simulink model "dsogi_pll_arch"  (R2023a)
settings: Solver=VariableStepAuto  StartTime=0.0  StopTime=10.0  RelTol=1e-3
settings Model: DataDictionary=dictionary.sldd  Creator=ASUSTUF  LastModifiedBy=ASUSTUF

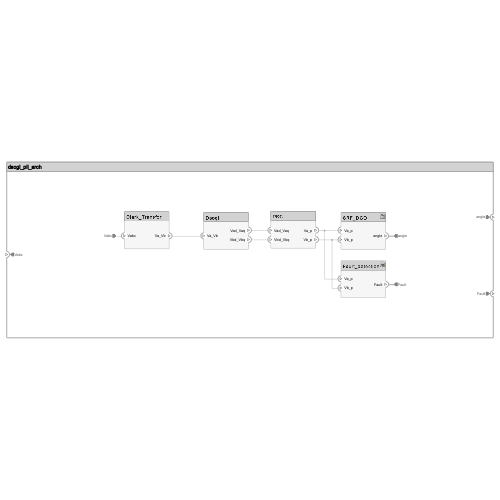
[thumbnail: Simulink's stored preview of the top-level diagram]
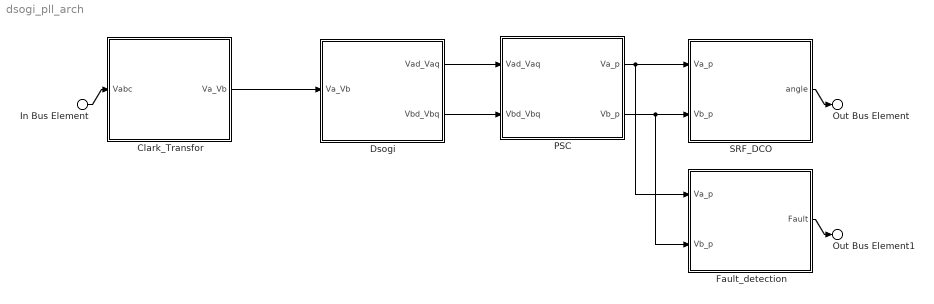
== system dsogi_pll_arch ==
  In Bus Element : Inport  PortName=Vabc
  Clark_Transfor : Subsystem
      settings: PortSchema="{\"entries\":[{\"content\":{\"headerSize\":26,\"margin\":15,\"minimumSpacing\":25,\"sides\":[{\"content\":{\"connectorIds\":[\"In1\"]},\"type\":\"ConnectorPlacement.EquallySpacedRectSide\",\"uuid\":\"d98255bb-0e2e-436f-ac53-b41bd6cffae4\"},{\"content\":{\"connectorIds\":[\"Out1\"],\"side\":\"RIGHT\"},\"type\":\"ConnectorPlacement.EquallySpacedRectSide\",\"uuid\":\"38fda810-9180-46c2-b72f-a00921e55bae\"},{\"content\":{\"side\":\"TOP\"},\"type\":\"ConnectorPlacement.EquallySpacedRectSide\",\"uuid\":\"74ae08d3-cfde-4772-a14d-4780a47b2df7\"}]},\"type\":\"ConnectorPlacement.EquallySpacedConnector\",\"uuid\":\"be157ddc-8a55-4c3c-90ba-55b865cce77e\"}],\"packageUris\":[\"http://schema.mathworks.com/mf0/Connector/R2020b\"],\"version\":\"1.0\"}"
  Dsogi : Subsystem
      settings: PortSchema="{\"entries\":[{\"content\":{\"headerSize\":26,\"margin\":15,\"minimumSpacing\":25,\"sides\":[{\"content\":{\"connectorIds\":[\"In1\"]},\"type\":\"ConnectorPlacement.EquallySpacedRectSide\",\"uuid\":\"d98255bb-0e2e-436f-ac53-b41bd6cffae4\"},{\"content\":{\"connectorIds\":[\"Out1\",\"Out2\"],\"side\":\"RIGHT\"},\"type\":\"ConnectorPlacement.EquallySpacedRectSide\",\"uuid\":\"38fda810-9180-46c2-b72f-a00921e55bae\"},{\"content\":{\"side\":\"TOP\"},\"type\":\"ConnectorPlacement.EquallySpacedRectSide\",\"uuid\":\"74ae08d3-cfde-4772-a14d-4780a47b2df7\"}]},\"type\":\"ConnectorPlacement.EquallySpacedConnector\",\"uuid\":\"be157ddc-8a55-4c3c-90ba-55b865cce77e\"}],\"packageUris\":[\"http://schema.mathworks.com/mf0/Connector/R2020b\"],\"version\":\"1.0\"}"
  Fault_detection : Subsystem
      settings: PortSchema="{\"entries\":[{\"content\":{\"headerSize\":26,\"margin\":15,\"minimumSpacing\":25,\"sides\":[{\"content\":{\"connectorIds\":[\"In1\",\"In2\"]},\"type\":\"ConnectorPlacement.EquallySpacedRectSide\",\"uuid\":\"d98255bb-0e2e-436f-ac53-b41bd6cffae4\"},{\"content\":{\"connectorIds\":[\"Out1\"],\"side\":\"RIGHT\"},\"type\":\"ConnectorPlacement.EquallySpacedRectSide\",\"uuid\":\"38fda810-9180-46c2-b72f-a00921e55bae\"},{\"content\":{\"side\":\"TOP\"},\"type\":\"ConnectorPlacement.EquallySpacedRectSide\",\"uuid\":\"74ae08d3-cfde-4772-a14d-4780a47b2df7\"}]},\"type\":\"ConnectorPlacement.EquallySpacedConnector\",\"uuid\":\"be157ddc-8a55-4c3c-90ba-55b865cce77e\"}],\"packageUris\":[\"http://schema.mathworks.com/mf0/Connector/R2020b\"],\"version\":\"1.0\"}"
  PSC : Subsystem
      settings: PortSchema="{\"entries\":[{\"content\":{\"headerSize\":26,\"margin\":15,\"minimumSpacing\":25,\"sides\":[{\"content\":{\"connectorIds\":[\"In2\",\"In1\"]},\"type\":\"ConnectorPlacement.EquallySpacedRectSide\",\"uuid\":\"d98255bb-0e2e-436f-ac53-b41bd6cffae4\"},{\"content\":{\"connectorIds\":[\"Out1\",\"Out2\"],\"side\":\"RIGHT\"},\"type\":\"ConnectorPlacement.EquallySpacedRectSide\",\"uuid\":\"38fda810-9180-46c2-b72f-a00921e55bae\"},{\"content\":{\"side\":\"TOP\"},\"type\":\"ConnectorPlacement.EquallySpacedRectSide\",\"uuid\":\"74ae08d3-cfde-4772-a14d-4780a47b2df7\"},{\"content\":{\"side\":\"BOTTOM\"},\"type\":\"ConnectorPlacement.EquallySpacedRectSide\",\"uuid\":\"92c08b77-8ee7-458d-a700-045080e1c0b7\"}]},\"type\":\"ConnectorPlacement.EquallySpacedConnector\",\"uuid\":\"be157ddc-8a55-4c3c-90ba-55b865cce77e\"}],\"packageUris\":[\"http://schema.mathworks.com/mf0/Connector/R2020b\"],\"version\":\"1.0\"}"
  SRF_DCO : Subsystem
      settings: PortSchema="{\"entries\":[{\"content\":{\"headerSize\":26,\"margin\":15,\"minimumSpacing\":25,\"sides\":[{\"content\":{\"connectorIds\":[\"In2\",\"In1\"]},\"type\":\"ConnectorPlacement.EquallySpacedRectSide\",\"uuid\":\"d98255bb-0e2e-436f-ac53-b41bd6cffae4\"},{\"content\":{\"connectorIds\":[\"Out1\"],\"side\":\"RIGHT\"},\"type\":\"ConnectorPlacement.EquallySpacedRectSide\",\"uuid\":\"38fda810-9180-46c2-b72f-a00921e55bae\"},{\"content\":{\"side\":\"TOP\"},\"type\":\"ConnectorPlacement.EquallySpacedRectSide\",\"uuid\":\"74ae08d3-cfde-4772-a14d-4780a47b2df7\"},{\"content\":{\"side\":\"BOTTOM\"},\"type\":\"ConnectorPlacement.EquallySpacedRectSide\",\"uuid\":\"8057ff04-3b7c-4155-979f-6ccb1b9af7cb\"}]},\"type\":\"ConnectorPlacement.EquallySpacedConnector\",\"uuid\":\"be157ddc-8a55-4c3c-90ba-55b865cce77e\"}],\"packageUris\":[\"http://schema.mathworks.com/mf0/Connector/R2020b\"],\"version\":\"1.0\"}"
  Out Bus Element : Outport  PortName=angle
  Out Bus Element1 : Outport  Port=2  PortName=Fault
  wires:
  Clark_Transfor/1(Va_Vb) -> Dsogi/1(Va_Vb)
  In Bus Element/1 -> Clark_Transfor/1(Vabc)
  Dsogi/1(Vad_Vaq) -> PSC/2(Vad_Vaq)
  Dsogi/2(Vbd_Vbq) -> PSC/1(Vbd_Vbq)
  PSC/1(Va_p) -> Fault_detection/1(Va_p), SRF_DCO/2(Va_p)
  PSC/2(Vb_p) -> Fault_detection/2(Vb_p), SRF_DCO/1(Vb_p)
  SRF_DCO/1(angle) -> Out Bus Element/1
  Fault_detection/1(Fault) -> Out Bus Element1/1

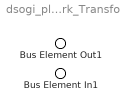
== system dsogi_pll_arch/Clark_Transfor ==
  Bus Element In1 : Inport  PortName=Vabc
  Bus Element Out1 : Outport  PortName=Va_Vb

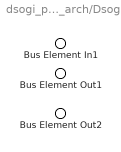
== system dsogi_pll_arch/Dsogi ==
  Bus Element In1 : Inport  PortName=Va_Vb
  Bus Element Out1 : Outport  PortName=Vad_Vaq
  Bus Element Out2 : Outport  Port=2  PortName=Vbd_Vbq

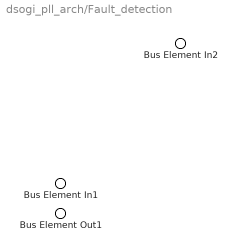
== system dsogi_pll_arch/Fault_detection ==
  Bus Element In2 : Inport  PortName=Va_p
  Bus Element In1 : Inport  Port=2  PortName=Vb_p
  Bus Element Out1 : Outport  PortName=Fault

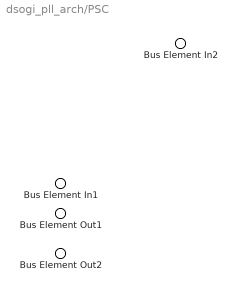
== system dsogi_pll_arch/PSC ==
  Bus Element In2 : Inport  PortName=Vbd_Vbq
  Bus Element In1 : Inport  Port=2  PortName=Vad_Vaq
  Bus Element Out1 : Outport  PortName=Va_p
  Bus Element Out2 : Outport  Port=2  PortName=Vb_p

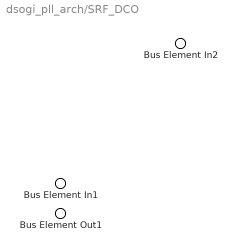
== system dsogi_pll_arch/SRF_DCO ==
  Bus Element In2 : Inport  PortName=Vb_p
  Bus Element In1 : Inport  Port=2  PortName=Va_p
  Bus Element Out1 : Outport  PortName=angle
